simulink model "controlador_imc"  (R2018a)
settings: Solver=VariableStepAuto  StartTime=0.0  StopTime=250  RelTol=1e-3
settings Model: Creator=root  LastModifiedBy=root

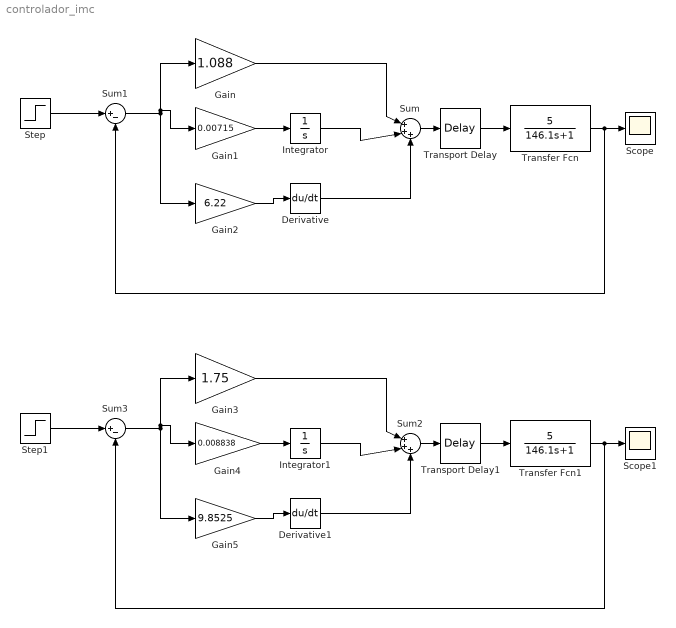
== system controlador_imc ==
  Derivative : Derivative
  Derivative1 : Derivative
  Gain : Gain  Gain=1.088
  Gain1 : Gain  Gain=0.00715
  Gain2 : Gain  Gain=6.22
  Gain3 : Gain  Gain=1.75
  Gain4 : Gain  Gain=0.008838
  Gain5 : Gain  Gain=9.8525
  Integrator : Integrator
  Integrator1 : Integrator
  Scope : Scope
  Scope1 : Scope
  Step : Step  Time=0  After=4  SampleTime=0
  Step1 : Step  Time=0  After=4  SampleTime=0
  Sum : Sum  Inputs=|+++
  Sum1 : Sum  Inputs=|+-
  Sum2 : Sum  Inputs=|+++
  Sum3 : Sum  Inputs=|+-
  Transfer Fcn : TransferFcn  Numerator=[5]  Denominator=[146.1 1]
  Transfer Fcn1 : TransferFcn  Numerator=[5]  Denominator=[146.1 1]
  Transport Delay : TransportDelay  DelayTime=11.9
  Transport Delay1 : TransportDelay  DelayTime=11.9
  wires:
  Gain/1 -> Sum/1
  Gain1/1 -> Integrator/1
  Gain2/1 -> Derivative/1
  Integrator/1 -> Sum/2
  Derivative/1 -> Sum/3
  Sum/1 -> Transport Delay/1
  Transport Delay/1 -> Transfer Fcn/1
  Step/1 -> Sum1/1
  Sum1/1 -> Gain1/1, Gain/1, Gain2/1
  Transfer Fcn/1 -> Scope/1, Sum1/2
  Step1/1 -> Sum3/1
  Integrator1/1 -> Sum2/2
  Gain3/1 -> Sum2/1
  Transport Delay1/1 -> Transfer Fcn1/1
  Sum2/1 -> Transport Delay1/1
  Sum3/1 -> Gain4/1, Gain3/1, Gain5/1
  Derivative1/1 -> Sum2/3
  Gain4/1 -> Integrator1/1
  Gain5/1 -> Derivative1/1
  Transfer Fcn1/1 -> Scope1/1, Sum3/2
